simulink model "Elevacion1"  (R2025b)
settings: Solver=VariableStepAuto  StartTime=0.0  StopTime=30.0  RelTol=1e-3
libraries: slpidlib x1, simulink x1
settings Model: Creator=alfon  LastModifiedBy=alfon

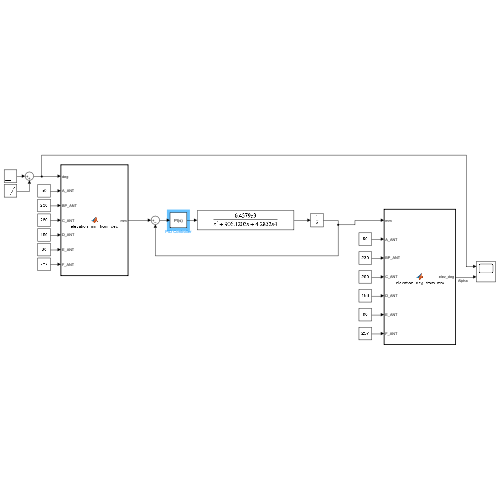
[thumbnail: Simulink's stored preview of the top-level diagram]
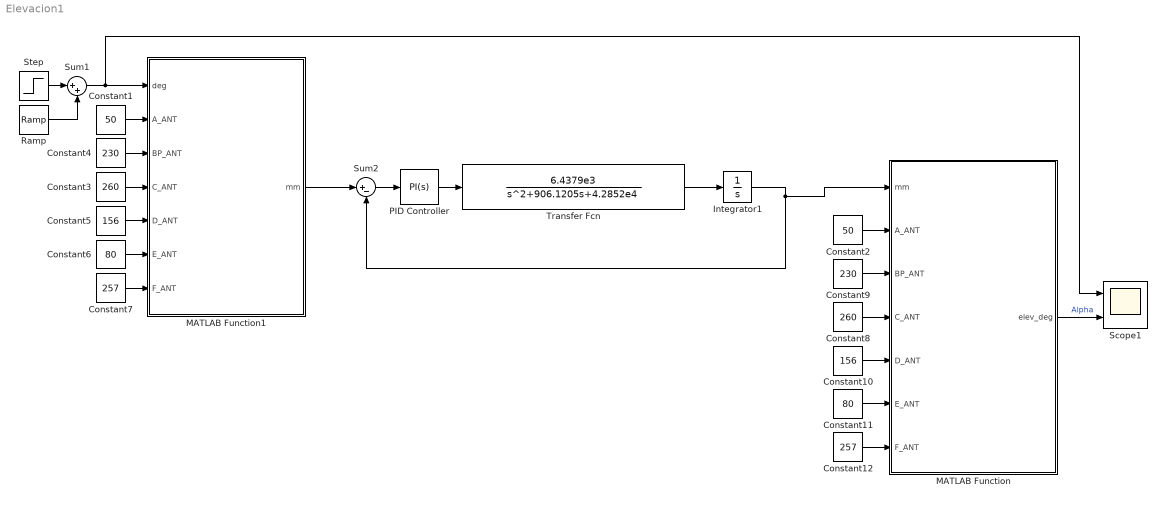
== system Elevacion1 ==
  Constant1 : Constant  Value=50
  Constant10 : Constant  Value=156
  Constant11 : Constant  Value=80
  Constant12 : Constant  Value=257
  Constant2 : Constant  Value=50
  Constant3 : Constant  Value=260
  Constant4 : Constant  Value=230
  Constant5 : Constant  Value=156
  Constant6 : Constant  Value=80
  Constant7 : Constant  Value=257
  Constant8 : Constant  Value=260
  Constant9 : Constant  Value=230
  Integrator1 : Integrator
  MATLAB Function : MATLAB Function  TreatAsAtomicUnit=on
  MATLAB Function1 : MATLAB Function  TreatAsAtomicUnit=on
  PID Controller : slpidlib/PID Controller  Controller=PI  Form=Parallel  TimeDomain=Continuous-time  UseExternalTs=off  SampleTime=-1  IntegratorMethod=Forward Euler  FilterMethod=Forward Euler  ControllerParametersSource=internal  P=5  I=0.05  UseKiTs=off  D=0  UseExternalDerivativeSource=off  N=100  UseFilter=on  TunerSelectOption=Transfer Function Based (PID Tuner App)  InitialConditionSource=internal  InitialConditionForIntegrator=0  InitialConditionForFilter=0  DifferentiatorICPrevScaledInput=0  ExternalReset=none  TrackingMode=off  Kt=1  LimitOutput=off  SatLimitsSource=internal  UpperSaturationLimit=inf  LowerSaturationLimit=-inf  LinearizeAsGain=on  AntiWindupMode=none  Kb=1  LimitIntegrator=off  UpperIntegratorSaturationLimit=inf  LowerIntegratorSaturationLimit=-inf  POutMin=[]  POutMax=[]  IOutMin=[]  IOutMax=[]  DOutMin=[]  DOutMax=[]  NOutMin=[]  NOutMax=[]  SumOutMin=[]  SumOutMax=[]  SaturationOutMin=[]  SaturationOutMax=[]  PParamMin=[]  PParamMax=[]  IParamMin=[]  IParamMax=[]  DParamMin=[]  DParamMax=[]  NParamMin=[]  NParamMax=[]  KbParamMin=[]  KbParamMax=[]  KtParamMin=[]  KtParamMax=[]  KbOutMin=[]  KbOutMax=[]  KtOutMin=[]  KtOutMax=[]  IntegratorOutMin=[]  IntegratorOutMax=[]  FilterOutMin=[]  FilterOutMax=[]  SumI1OutMin=[]  SumI1OutMax=[]  SumI2OutMin=[]  SumI2OutMax=[]  SumI3OutMin=[]  SumI3OutMax=[]  SumI4OutMin=[]  SumI4OutMax=[]  SumDOutMin=[]  SumDOutMax=[]  DifferentiatorOutMin=[]  DifferentiatorOutMax=[]  FilterDiffOutCoefMin=[]  FilterDiffOutCoefMax=[]  ReciprocalOutMin=[]  ReciprocalOutMax=[]  SumDenOutMin=[]  SumDenOutMax=[]  SumNumOutMin=[]  SumNumOutMax=[]  DivideOutMin=[]  DivideOutMax=[]  UdiffTsProdOutMin=[]  UdiffTsProdOutMax=[]  NTsProdOutMin=[]  NTsProdOutMax=[]  UintegralTsProdOutMin=[]  UintegralTsProdOutMax=[]  UngainTsProdOutMin=[]  UngainTsProdOutMax=[]  ClampingZeroOutDataTypeStr=Inherit: Inherit via back propagation  ClampingZeroOutMin=[]  ClampingZeroOutMax=[]  FilterDenConstantOutDataTypeStr=Inherit: Inherit via back propagation  FilterDenConstantOutMin=[]  FilterDenConstantOutMax=[]  PCopyOutDataTypeStr=Inherit: Inherit via back propagation  PCopyOutMin=[]  PCopyOutMax=[]  NCopyOutDataTypeStr=Inherit: Inherit via back propagation  NCopyOutMin=[]  NCopyOutMax=[]  IntegratorContinuousStateAttributes=''  IntegratorStateMustResolveToSignalObject=off  IntegratorRTWStateStorageClass=Auto  FilterContinuousStateAttributes=''  FilterStateMustResolveToSignalObject=off  FilterRTWStateStorageClass=Auto  ParallelPVariant=InternalParameters  IdealPVariant=Disabled  IVariant=InternalParameters  DVariant=Disabled  IntegratorVariant=Continuous  SatVariant=Disabled  AWVariant=Passthrough  PCopyVariant=Disabled  TRVariant=Disabled  FdbkBlocksVariant=Forward  IdealPFdbkVariant=Disabled  SatFdbkVariant=Disabled  DerivativeFilterVariant=Disabled  NVariant=Disabled  NCopyVariant=Disabled_SignalSpec  FilterICVariant=Disabled  IntegratorICVariant=InternalICs  ExternalResetVariant=Disabled  TRSumVariant=Passthrough  SumFdbkVariant=Disabled  SumVariant=Sum_PI  TsampFilterVariant=InternalTs  TsampNgainVariant=Passthrough  TsampIntegralVariant=Disabled_SignalSpec  ExternalSaturationOutDataTypeStr=Inherit: Same as second input  DerivativeSourceVariant=Disabled  PreIntVariant=InternalPreInt
  Ramp : simulink/Sources/Ramp  slope=-0.1  start=0  InitialOutput=0
  Scope1 : Scope  NumInputPorts=2
      settings: ActiveDisplayYMinimum=49.318304712800348  ActiveDisplayYMaximum=102.78214021428158
  Step : Step  Time=0  After=60  SampleTime=0
  Sum1 : Sum  Inputs=|++
  Sum2 : Sum  Inputs=|+-
  Transfer Fcn : TransferFcn  Numerator=[6.4379e3]  Denominator=[1,906.1205,4.2852e4]
  wires:
  Constant11/1 -> MATLAB Function/6(E_ANT)
  Constant4/1 -> MATLAB Function1/3(BP_ANT)
  Step/1 -> Sum1/1
  Constant8/1 -> MATLAB Function/4(C_ANT)
  Constant3/1 -> MATLAB Function1/4(C_ANT)
  Constant6/1 -> MATLAB Function1/6(E_ANT)
  MATLAB Function/1(elev_deg) -> Scope1/2  "Alpha"
  Constant1/1 -> MATLAB Function1/2(A_ANT)
  Constant5/1 -> MATLAB Function1/5(D_ANT)
  Constant7/1 -> MATLAB Function1/7(F_ANT)
  Constant12/1 -> MATLAB Function/7(F_ANT)
  Sum1/1 -> Scope1/1, MATLAB Function1/1(deg)
  Constant2/1 -> MATLAB Function/2(A_ANT)
  Ramp/1 -> Sum1/2
  Constant9/1 -> MATLAB Function/3(BP_ANT)
  Constant10/1 -> MATLAB Function/5(D_ANT)
  MATLAB Function1/1(mm) -> Sum2/1
  Sum2/1 -> PID Controller/1
  PID Controller/1 -> Transfer Fcn/1
  Transfer Fcn/1 -> Integrator1/1
  Integrator1/1 -> Sum2/2, MATLAB Function/1(mm)

== matlab function Elevacion1/MATLAB Function1 ==
  data: deg input; mm output; A_ANT input; BP_ANT input; C_ANT input; D_ANT input; E_ANT input; F_ANT input
function mm = elevation_mm_from_deg(deg, A_ANT, BP_ANT, C_ANT, D_ANT, E_ANT, F_ANT)
A_CONST = 3*pi/2 - atan2(C_ANT, D_ANT) - atan2(F_ANT, E_ANT);

B_CONST = 2 * sqrt( (F_ANT^2 + E_ANT^2) * (D_ANT^2 + C_ANT^2) );

C_CONST = F_ANT^2 + E_ANT^2 + D_ANT^2 + C_ANT^2 - A_ANT^2;

DEG_TO_RAD = pi/180;

mm = sqrt(C_CONST - B_CONST * cos(A_CONST - DEG_TO_RAD * deg)) - BP_ANT;

end

== matlab function Elevacion1/MATLAB Function ==
  data: mm input; elev_deg output; A_ANT input; BP_ANT input; C_ANT input; D_ANT input; E_ANT input; F_ANT input
function elev_deg = elevation_deg_from_mm(mm, A_ANT, BP_ANT, C_ANT, D_ANT, E_ANT, F_ANT)

A_CONST = 3*pi/2 - atan2(C_ANT, D_ANT) - atan2(F_ANT, E_ANT);

B_CONST = 2 * sqrt((F_ANT^2 + E_ANT^2) * (D_ANT^2 + C_ANT^2));

C_CONST = F_ANT^2 + E_ANT^2 + D_ANT^2 + C_ANT^2 - A_ANT^2;

elev_deg = (A_CONST - acos((C_CONST - (BP_ANT + mm)^2) / B_CONST)) * 180/pi;
end
